simulink library "library_GPSPackaging"  (R2024a)
settings: Solver=VariableStepAuto  StartTime=0.0  StopTime=10.0  RelTol=1e-3
libraries: library_IMUPackagingSFunc x1
settings Model: Creator=tommy  LastModifiedBy=tommy

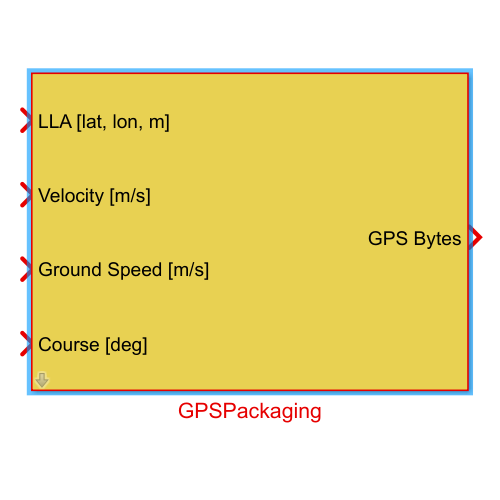
[thumbnail: Simulink's stored preview of the top-level diagram]
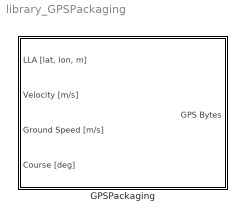
== system library_GPSPackaging ==
  GPSPackaging : Subsystem
      mask help: Default Mask

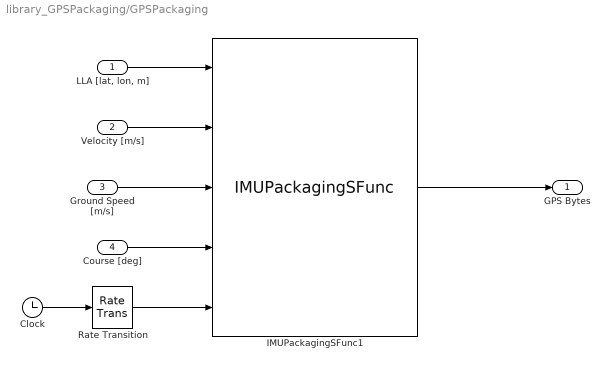
== system library_GPSPackaging/GPSPackaging ==
  "LLA [lat, lon, m]" : Inport
  Velocity [m/s] : Inport  Port=2
  Ground Speed [m/s] : Inport  Port=3
  Course [deg] : Inport  Port=4
  Clock : Clock
  IMUPackagingSFunc1 : library_IMUPackagingSFunc/IMUPackagingSFunc
  Rate Transition : RateTransition  OutPortSampleTimeOpt=Inherit
  GPS Bytes : Outport
  wires:
  Rate Transition/1 -> IMUPackagingSFunc1/5
  Clock/1 -> Rate Transition/1
  Course [deg]/1 -> IMUPackagingSFunc1/4
  Ground Speed [m/s]/1 -> IMUPackagingSFunc1/3
  Velocity [m/s]/1 -> IMUPackagingSFunc1/2
  "LLA [lat, lon, m]"/1 -> IMUPackagingSFunc1/1
  IMUPackagingSFunc1/1 -> GPS Bytes/1
